simulink model "Simulation_File"  (R2017a)
settings: Solver=VariableStepAuto  StartTime=0.0  StopTime=50  FixedStep=Tsg  MaxStep=1e-3  RelTol=1e-3  EnableMultiTasking=on
InitFcn:
  | load('Wind_Perfil.mat')
  | 
  | Tsg=(1/5000);
  | TsPID=(1/5000);
  | TsWidfCV=0.01;
  | Ts=(1/5000);
  | 
  | %Parametros del convertidor
  | RD=0.01;
  | RQ=0.001;
  | RCi=0.01;
  | %RCi=0.1;
  | %RCi=1;
  | VD=0.7;
  | RL=0.1;
  | Ci=470e-6;
  | L=0.08;
  | Vdc_link=190.1681;
  | %Fs=5e3/1;
  | %Ts=1/Fs;
  | 
  | 
  | 
  | 
  | %% Battery Parameters
  | n_series = 50; % Number of series connected cells
  | n_parallel = 2; % Number of parallel branches
  | SOC_init = 0.5; % initial SOC
  | 
  | cell_cap = 6.5; % Cell capacitance
  | pack_cap = cell_cap * n_parallel; % Pack capacitance
  | 
  | cell_ConstI = 1.3; % Target constant charging current for each cell
  | cell_ConstV = 4.1; % Target constant charging voltage for each cell
  | 
  | ConstI = cell_ConstI * n_parallel; % Target constant charging current
  | ConstV = cell_ConstV * n_series; % Target constant charging voltage
  | 
  | MAX_SOC = 0.97; % State of charge when battery charging is stopped
  | 
  | %Parametros relacionados a sensado de corriente
  | G=100*1;
  | RG=1e3;
  | Rf=((G-1)*RG)/2;
  | DCR=RL;
  | Rcs=10e3;
  | Ccs=L/(DCR*Rcs);
undefined symbols (not defined in the file or in its folder): plecs
libraries: pil_lib x1
Description:
  | Software-in-the-Loop Code Verification
settings Model: ExtModeTrigDuration=10  ExtModeAutoUpdateStatusClock=off  Creator=The MathWorks, Inc.  LastModifiedBy=David R. LF
settings DataIOCC: SaveFormat=Array  SignalLogging=off  ReturnWorkspaceOutputs=on  SignalLoggingName=sigsOut
settings OptimizationCC: UseDivisionForNetSlopeComputation=UseDivisionForReciprocalsOfIntegersOnly  DefaultUnderspecifiedDataType=single  EnhancedBackFolding=on  BooleansAsBitfields=on  PassReuseOutputArgsAs=Individual arguments  ExpressionDepthLimit=2147483647  StateBitsets=on  DataBitsets=on  ZeroExternalMemoryAtStartup=off  NoFixptDivByZeroProtection=on  EfficientFloat2IntCast=on  LifeSpan=1  MaxStackSize=2560
settings DebuggingCC: CheckExecutionContextPreStartOutputMsg=on  CheckExecutionContextRuntimeOutputMsg=on  FcnCallInpInsideContextMsg=warning  AllowSymbolicDim=off  StateNameClashWarn=warning  StrictBusMsg=ErrorOnBusTreatedAsVector  SFUnexpectedBacktrackingDiag=warning  SFNoUnconditionalDefaultTransitionDiag=warning  SFExecutionAtInitializationDiag=none
settings HardwareCC: ProdBitPerPointer=32  ProdBitPerSizeT=32  ProdBitPerPtrDiffT=32  ProdLargestAtomicInteger=Long  ProdLargestAtomicFloat=Double  ProdWordSize=32  ProdLongLongMode=on  ProdHWDeviceType=ARM Compatible->ARM Cortex  TargetBitPerPointer=64  TargetBitPerSizeT=64  TargetBitPerPtrDiffT=64  TargetLongLongMode=on  TargetIntDivRoundTo=Zero  TargetEndianess=LittleEndian  TargetWordSize=64  TargetHWDeviceType=Generic->MATLAB Host Computer
settings ModelReferenceCC: PropagateSignalLabelsOutOfModel=off
settings SFSimCC: MATLABDynamicMemAlloc=off
settings RTWCC: SystemTargetFile=ert.tlc  HardwareBoard=TI Concerto F28M35x (ARM Cortex-M3)  TemplateMakefile=ert_default_tmf  Description=Embedded Coder  GenerateReport=on  RTWVerbose=off  Toolchain=Texas Instruments Code Composer Studio v6 (ARM)  IncludeHyperlinkInReport=on  CreateSILPILBlock=PIL  GenerateTraceInfo=on  GenerateTraceReport=on  GenerateTraceReportSl=on  GenerateTraceReportSf=on  GenerateTraceReportEml=on  GenerateCodeMetricsReport=on
settings CodeAppCC: ForceParamTrailComments=on  IgnoreCustomStorageClasses=off  IgnoreTestpoints=on  SimulinkDataObjDesc=on  CustomSymbolStrGlobalVar=rt$N$M  CustomSymbolStrType=$N$M  CustomSymbolStrFcn=$N$M$F  CustomSymbolStrMacro=$N$M  InsertBlockDesc=on  InternalIdentifier=Classic
settings ERTTargetCC: UtilityFuncGeneration=Shared location  MultiwordLength=2048  IncludeMdlTerminateFcn=off  CombineSignalStateStructs=on  SupportNonFinite=off  SupportContinuousTime=on  SupportVariableSizeSignals=on  ERTFilePackagingFormat=CompactWithDataFile  ConvertIfToSwitch=off  SuppressUnreachableDefaultCases=off
settings ConfigComp: CovMetricSettings=dw  CovHtmlReporting=on  CovSaveCumulativeToWorkspaceVar=on  CovSaveSingleToWorkspaceVar=on  CovExternalEMLEnable=off  CovSFcnEnable=off

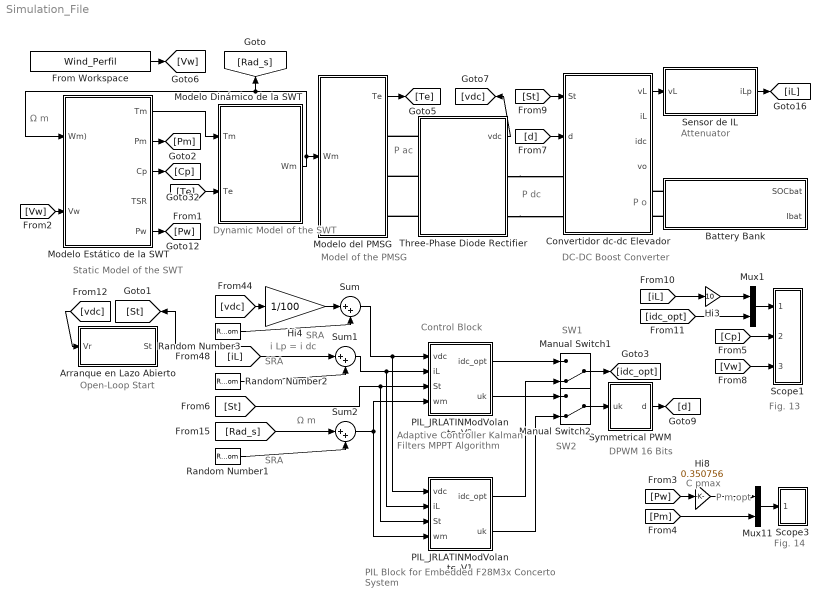
== system Simulation_File ==
  note: DPWM
      | 16 Bits
  note: i Lp = i dc
  note: Adaptive Controller
      | Kalman Filters
      | MPPT Algorithm
  note: Attenuator
  note: Open-Loop
      | Start
  note: DC-DC
      | Boost Converter
  note: P ac
  note: Model of
      | the PMSG
  note: Static Model
      | of the SWT
  note: Dynamic Model
      | of the SWT
  note: Ω m
  note: P dc
  note: P o
  note: SRA
  note: SRA
  note: Ω m
  note: SRA
  note: C pmax
  note: P m,opt
  note: Fig. 13
  note: Fig. 14
  note: PIL Block for Embedded F28M3x
      | Concerto System
  note: Control Block
  note: SW1
  note: SW2
  Arranque en Lazo Abierto : Subsystem  LoadFcn=plecs('sl', 200);  InitFcn=plecs('sl', 214);  StartFcn=plecs('sl', 208);  StopFcn=plecs('sl', 209);  mask(PlecsCircuit){PLECSData=<binary blob, 2632 chars, not shown>}
      mask prompts: PLECSData "PLECS Data (Do not delete or modify!)"
      mask init:
      | % PLACE CUSTOM INITIALIZATIONS ABOVE
      | % DO NOT REMOVE
      | plecs('sl', 215);
      | % DO NOT REMOVE
      settings: CopyFcn=plecs('sl', 203);  DeleteFcn=plecs('sl', 205);  UndoDeleteFcn=plecs('sl', 206);  PreSaveFcn=plecs('sl', 211);  PostSaveFcn=plecs('sl', 201);  NameChangeFcn=plecs('sl', 210);  DestroyFcn=plecs('sl', 207);  PreCopyFcn=plecs('sl', 216);  OpenFcn=plecs('sl', 202);  ErrorFcn=plerrorfcn
      mask Help: web(['file:///' fullfile(plecsdoc, 'creatingacircuit.html')])
      mask Display: disp('PLECS\nCircuit')
  Battery Bank : Subsystem  LoadFcn=plecs('sl', 200);  InitFcn=plecs('sl', 214);  StartFcn=plecs('sl', 208);  StopFcn=plecs('sl', 209);  mask(PlecsCircuit){PLECSData=<binary blob, 6620 chars, not shown>}
      mask prompts: PLECSData "PLECS Data (Do not delete or modify!)"
      mask init:
      | % PLACE CUSTOM INITIALIZATIONS ABOVE
      | % DO NOT REMOVE
      | plecs('sl', 215);
      | % DO NOT REMOVE
      settings: CopyFcn=plecs('sl', 203);  DeleteFcn=plecs('sl', 205);  UndoDeleteFcn=plecs('sl', 206);  PreSaveFcn=plecs('sl', 211);  PostSaveFcn=plecs('sl', 201);  NameChangeFcn=plecs('sl', 210);  DestroyFcn=plecs('sl', 207);  PreCopyFcn=plecs('sl', 216);  OpenFcn=plecs('sl', 202);  ErrorFcn=plerrorfcn
      mask Help: web(['file:///' fullfile(plecsdoc, 'creatingacircuit.html')])
      mask Display: disp('PLECS\nCircuit')
  Convertidor dc-dc Elevador : Subsystem  LoadFcn=plecs('sl', 200);  InitFcn=plecs('sl', 214);  StartFcn=plecs('sl', 208);  StopFcn=plecs('sl', 209);  mask(PlecsCircuit){PLECSData=<binary blob, 2184 chars, not shown>}
      mask prompts: PLECSData "PLECS Data (Do not delete or modify!)"
      mask init:
      | % PLACE CUSTOM INITIALIZATIONS ABOVE
      | % DO NOT REMOVE
      | plecs('sl', 215);
      | % DO NOT REMOVE
      settings: CopyFcn=plecs('sl', 203);  DeleteFcn=plecs('sl', 205);  UndoDeleteFcn=plecs('sl', 206);  PreSaveFcn=plecs('sl', 211);  PostSaveFcn=plecs('sl', 201);  NameChangeFcn=plecs('sl', 210);  DestroyFcn=plecs('sl', 207);  PreCopyFcn=plecs('sl', 216);  OpenFcn=plecs('sl', 202);  ErrorFcn=plerrorfcn
      mask Help: web(['file:///' fullfile(plecsdoc, 'creatingacircuit.html')])
      mask Display: disp('PLECS\nCircuit')
  From Workspace : FromWorkspace  VariableName=Wind_Perfil  SampleTime=1e-3
  Hi3 : Gain  Gain=10
  Hi4 : Gain  Gain=1/100
  Hi8 : Gain  Gain=0.350756
  Manual Switch1 : ManualSwitch  CurrentSetting=0
  Manual Switch2 : ManualSwitch  CurrentSetting=0
  Modelo del PMSG : Subsystem  LoadFcn=plecs('sl', 200);  InitFcn=plecs('sl', 214);  StartFcn=plecs('sl', 208);  StopFcn=plecs('sl', 209);  mask(PlecsCircuit){PLECSData=<binary blob, 5964 chars, not shown>}
      mask prompts: PLECSData "PLECS Data (Do not delete or modify!)"
      mask init:
      | % PLACE CUSTOM INITIALIZATIONS ABOVE
      | % DO NOT REMOVE
      | plecs('sl', 215);
      | % DO NOT REMOVE
      settings: CopyFcn=plecs('sl', 203);  DeleteFcn=plecs('sl', 205);  UndoDeleteFcn=plecs('sl', 206);  PreSaveFcn=plecs('sl', 211);  PostSaveFcn=plecs('sl', 201);  NameChangeFcn=plecs('sl', 210);  DestroyFcn=plecs('sl', 207);  PreCopyFcn=plecs('sl', 216);  OpenFcn=plecs('sl', 202);  ErrorFcn=plerrorfcn
      mask Help: web(['file:///' fullfile(plecsdoc, 'creatingacircuit.html')])
      mask Display: disp('PLECS\nCircuit')
  "Modelo Dinámico de la SWT " : Subsystem  LoadFcn=plecs('sl', 200);  InitFcn=plecs('sl', 214);  StartFcn=plecs('sl', 208);  StopFcn=plecs('sl', 209);  mask(PlecsCircuit){PLECSData=<binary blob, 2232 chars, not shown>}
      mask prompts: PLECSData "PLECS Data (Do not delete or modify!)"
      mask init:
      | % PLACE CUSTOM INITIALIZATIONS ABOVE
      | % DO NOT REMOVE
      | plecs('sl', 215);
      | % DO NOT REMOVE
      settings: CopyFcn=plecs('sl', 203);  DeleteFcn=plecs('sl', 205);  UndoDeleteFcn=plecs('sl', 206);  PreSaveFcn=plecs('sl', 211);  PostSaveFcn=plecs('sl', 201);  NameChangeFcn=plecs('sl', 210);  DestroyFcn=plecs('sl', 207);  PreCopyFcn=plecs('sl', 216);  OpenFcn=plecs('sl', 202);  ErrorFcn=plerrorfcn
      mask Help: web(['file:///' fullfile(plecsdoc, 'creatingacircuit.html')])
      mask Display: disp('PLECS\nCircuit')
  "Modelo Estático de la SWT " : Subsystem  LoadFcn=plecs('sl', 200);  InitFcn=plecs('sl', 214);  StartFcn=plecs('sl', 208);  StopFcn=plecs('sl', 209);  mask(PlecsCircuit){PLECSData=<binary blob, 3544 chars, not shown>}
      mask prompts: PLECSData "PLECS Data (Do not delete or modify!)"
      mask init:
      | % PLACE CUSTOM INITIALIZATIONS ABOVE
      | % DO NOT REMOVE
      | plecs('sl', 215);
      | % DO NOT REMOVE
      settings: CopyFcn=plecs('sl', 203);  DeleteFcn=plecs('sl', 205);  UndoDeleteFcn=plecs('sl', 206);  PreSaveFcn=plecs('sl', 211);  PostSaveFcn=plecs('sl', 201);  NameChangeFcn=plecs('sl', 210);  DestroyFcn=plecs('sl', 207);  PreCopyFcn=plecs('sl', 216);  OpenFcn=plecs('sl', 202);  ErrorFcn=plerrorfcn
      mask Help: web(['file:///' fullfile(plecsdoc, 'creatingacircuit.html')])
      mask Display: disp('PLECS\nCircuit')
  Mux1 : Mux  Inputs=2
  Mux11 : Mux  Inputs=2
  PIL_JRLATINModVolante_V1 : Subsystem  DialogController=pil_create_dialog  LoadFcn=|
      | try
      |    if ~strcmp(rtw.pil.getPILVersion, '6.12 (R2017a)_12')
      |       set_param(gcb, 'DialogController', '');
      |       set_param(gcb, 'DialogControllerArgs', '');
      |    end
      | catch e
      |       set_param(gcb, 'DialogController', '');
      |       set_param(gcb, 'DialogControllerArgs', '');
      | end
      mask help: PIL:pil:XILBlockMaskDesc
      mask Display: disp('PIL');
  PIL_JRLATINModVolante_V2 : Subsystem
  Random Number1 : RandomNumber  Variance=10*1  SampleTime=1e-3
  Random Number2 : RandomNumber  Variance=0.001*1  SampleTime=1e-3
  Random Number3 : RandomNumber  Variance=0.001*1  SampleTime=1e-3
  Scope1 : Subsystem  LoadFcn=plecs('sl', 300);  InitFcn=plecs('sl', 314);  StartFcn=plecs('sl', 308);  StopFcn=plecs('sl', 309);  mask{Settings=<binary blob, 1632 chars, not shown>}
      mask init:
      | plecs('sl', 315);
      settings: CopyFcn=plecs('sl', 303);  DeleteFcn=plecs('sl', 305);  UndoDeleteFcn=plecs('sl', 306);  PreSaveFcn=plecs('sl', 311);  NameChangeFcn=plecs('sl', 310);  DestroyFcn=plecs('sl', 307);  OpenFcn=plecs('sl', 302);  ErrorFcn=plerrorfcn
      mask Display: plot([0.1 0.9 0.9 0.1 0.1], [0.9 0.9 0.5 0.5 0.9])
  Scope3 : Subsystem  LoadFcn=plecs('sl', 300);  InitFcn=plecs('sl', 314);  StartFcn=plecs('sl', 308);  StopFcn=plecs('sl', 309);  mask{Settings=<binary blob, 1220 chars, not shown>}
      mask init:
      | plecs('sl', 315);
      settings: CopyFcn=plecs('sl', 303);  DeleteFcn=plecs('sl', 305);  UndoDeleteFcn=plecs('sl', 306);  PreSaveFcn=plecs('sl', 311);  NameChangeFcn=plecs('sl', 310);  DestroyFcn=plecs('sl', 307);  OpenFcn=plecs('sl', 302);  ErrorFcn=plerrorfcn
      mask Display: plot([0.1 0.9 0.9 0.1 0.1], [0.9 0.9 0.5 0.5 0.9])
  Sensor de IL : Subsystem  LoadFcn=plecs('sl', 200);  InitFcn=plecs('sl', 214);  StartFcn=plecs('sl', 208);  StopFcn=plecs('sl', 209);  mask(PlecsCircuit){PLECSData=<binary blob, 3020 chars, not shown>}
      mask prompts: PLECSData "PLECS Data (Do not delete or modify!)"
      mask init:
      | % PLACE CUSTOM INITIALIZATIONS ABOVE
      | % DO NOT REMOVE
      | plecs('sl', 215);
      | % DO NOT REMOVE
      settings: CopyFcn=plecs('sl', 203);  DeleteFcn=plecs('sl', 205);  UndoDeleteFcn=plecs('sl', 206);  PreSaveFcn=plecs('sl', 211);  PostSaveFcn=plecs('sl', 201);  NameChangeFcn=plecs('sl', 210);  DestroyFcn=plecs('sl', 207);  PreCopyFcn=plecs('sl', 216);  OpenFcn=plecs('sl', 202);  ErrorFcn=plerrorfcn
      mask Help: web(['file:///' fullfile(plecsdoc, 'creatingacircuit.html')])
      mask Display: disp('PLECS\nCircuit')
  Sum : Sum  Inputs=|++
  Sum1 : Sum  Inputs=|++
  Sum2 : Sum  Inputs=|++
  Symmetrical PWM : Subsystem  AncestorBlock=plecslib_extras2/Modulators/Symmetrical PWM  mask(Symmetrical PWM){sampling=Natural (carrier starts with 0), fc=5000, offset=0, input_limits=[0 65535], output_values=[0 1]}
      mask prompts: fc "Carrier frequency (Hz):"; offset "Carrier offset (p.u.):"; input_limits "Input limits [min max]:"; output_values "Output values [off on]:"
      mask help: PWM generator with a symmetrical triangular carrier. If the input is a vector, the output is also a vector of the same width.
      mask init:
      | if numel(fc)>1 || fc<=0,
      |   error('Carrier frequency must be a positive scalar.');
      | end
      | if numel(offset)>1 || offset<0 || offset>=1,
      |   error('Carrier offset must be a scalar in the range [0; 1/fc[.');
      | end
      | if sampling == 1,
      |   offset = mod(offset+.75, 1);
      | end
      | 
      | si = [.5 mod(offset, .5)]/fc;
      mask Help: eval('plecs(''help'', ''symmetricalpwm.html'')')
      mask TypeOptions sampling: Natural (carrier starts with 0) | Natural (carrier starts with 1) | Regular (double edge) | Regular (single edge)
  Three-Phase Diode Rectifier : Subsystem  LoadFcn=plecs('sl', 200);  InitFcn=plecs('sl', 214);  StartFcn=plecs('sl', 208);  StopFcn=plecs('sl', 209);  mask(PlecsCircuit){PLECSData=<binary blob, 1820 chars, not shown>}
      mask prompts: PLECSData "PLECS Data (Do not delete or modify!)"
      mask init:
      | % PLACE CUSTOM INITIALIZATIONS ABOVE
      | % DO NOT REMOVE
      | plecs('sl', 215);
      | % DO NOT REMOVE
      settings: CopyFcn=plecs('sl', 203);  DeleteFcn=plecs('sl', 205);  UndoDeleteFcn=plecs('sl', 206);  PreSaveFcn=plecs('sl', 211);  PostSaveFcn=plecs('sl', 201);  NameChangeFcn=plecs('sl', 210);  DestroyFcn=plecs('sl', 207);  PreCopyFcn=plecs('sl', 216);  OpenFcn=plecs('sl', 202);  ErrorFcn=plerrorfcn
      mask Help: web(['file:///' fullfile(plecsdoc, 'creatingacircuit.html')])
      mask Display: disp('PLECS\nCircuit')
  wires:
  Modelo del PMSG/1(Te) -> [Te]
  [St] -> Convertidor dc-dc Elevador/1(St)
  [d] -> Convertidor dc-dc Elevador/2(d)
  [Te] -> "Modelo Dinámico de la SWT "/2(Te)
  Three-Phase Diode Rectifier/1(vdc) -> [vdc]
  Sum/1 -> PIL_JRLATINModVolante_V1/1(vdc), PIL_JRLATINModVolante_V2/1(vdc)
  Sum1/1 -> PIL_JRLATINModVolante_V1/2(iL), PIL_JRLATINModVolante_V2/2(iL)
  [vdc] -> Arranque en Lazo Abierto/1(Vr)
  Arranque en Lazo Abierto/1(St) -> [St]
  [iL] -> Sum1/1
  Random Number2/1 -> Sum1/2
  Random Number3/1 -> Sum/2
  Sensor de IL/1(iLp) -> [iL]
  [St] -> PIL_JRLATINModVolante_V1/3(St), PIL_JRLATINModVolante_V2/3(St)
  "Modelo Estático de la SWT "/1(Tm) -> "Modelo Dinámico de la SWT "/1(Tm)
  "Modelo Dinámico de la SWT "/1(Wm) -> "Modelo Estático de la SWT "/1(Wm)), [Rad_s], Modelo del PMSG/1(Wm)
  [Vw] -> "Modelo Estático de la SWT "/2(Vw)
  Symmetrical PWM/1(d) -> [d]
  [Rad_s] -> Sum2/1
  Random Number1/1 -> Sum2/2
  Sum2/1 -> PIL_JRLATINModVolante_V1/4(wm), PIL_JRLATINModVolante_V2/4(wm)
  From Workspace/1 -> [Vw]
  Hi4/1 -> Sum/1
  [vdc] -> Hi4/1
  Convertidor dc-dc Elevador/1(vL) -> Sensor de IL/1(vL)
  "Modelo Estático de la SWT "/5(Pw) -> [Pw]
  [Pw] -> Hi8/1
  Hi8/1 -> Mux11/1
  Mux11/1 -> Scope3/1(1)
  "Modelo Estático de la SWT "/2(Pm) -> [Pm]
  [Pm] -> Mux11/2
  "Modelo Estático de la SWT "/3(Cp) -> [Cp]
  [Cp] -> Scope1/2(2)
  [Vw] -> Scope1/3(3)
  Mux1/1 -> Scope1/1(1)
  [idc_opt] -> Mux1/2
  [iL] -> Hi3/1
  Hi3/1 -> Mux1/1
  Manual Switch2/1 -> Symmetrical PWM/1(uk)
  PIL_JRLATINModVolante_V2/2(uk) -> Manual Switch2/1
  PIL_JRLATINModVolante_V2/1(idc_opt) -> Manual Switch1/1
  Manual Switch1/1 -> [idc_opt]
  PIL_JRLATINModVolante_V1/2(uk) -> Manual Switch2/2
  PIL_JRLATINModVolante_V1/1(idc_opt) -> Manual Switch1/2
  connections:
  Battery Bank/LConn1 -- Convertidor dc-dc Elevador/RConn1
  Three-Phase Diode Rectifier/LConn3 -- Modelo del PMSG/RConn3
  Three-Phase Diode Rectifier/LConn1 -- Modelo del PMSG/RConn1
  Three-Phase Diode Rectifier/RConn2 -- Convertidor dc-dc Elevador/LConn2
  Three-Phase Diode Rectifier/LConn2 -- Modelo del PMSG/RConn2
  Three-Phase Diode Rectifier/RConn1 -- Convertidor dc-dc Elevador/LConn1
  Battery Bank/LConn2 -- Convertidor dc-dc Elevador/RConn2

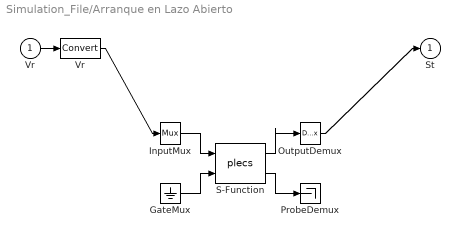
== system Simulation_File/Arranque en Lazo Abierto ==
  Vr : Inport  PortDimensions=1
  " GateMux " : Ground
  " InputMux " : Mux  Inputs=[ 1 ]
  " OutputDemux " : Demux  Outputs=[ 1 ]
  " ProbeDemux " : Terminator
  " S-Function " : S-Function  FunctionName=plecs  SFunctionDeploymentMode=off  EnableBusSupport=off
  " Vr " : DataTypeConversion  SaturateOnIntegerOverflow=on  RndMeth=Zero
  St : Outport  PortDimensions=1
  wires:
  " S-Function "/1 -> " OutputDemux "/1
  " InputMux "/1 -> " S-Function "/1
  " GateMux "/1 -> " S-Function "/2
  " S-Function "/2 -> " ProbeDemux "/1
  Vr/1 -> " Vr "/1
  " Vr "/1 -> " InputMux "/1
  " OutputDemux "/1 -> St/1

== system Simulation_File/Battery Bank ==
  +Vbat : PMIOPort  Port=1  Side=Left
  -Vbat : PMIOPort  Port=2  Side=Left
  SOCbat : Outport  PortDimensions=1
  Ibat : Outport  Port=2  PortDimensions=1
  wires:
  [PlecsSlave0Output1] -> SOCbat/1
  [PlecsSlave0Output2] -> Ibat/1

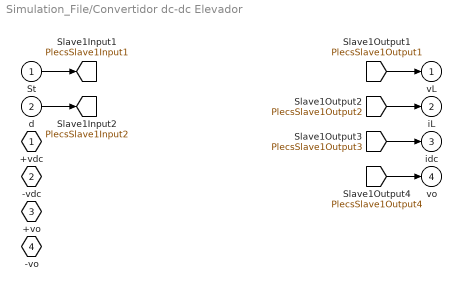
== system Simulation_File/Convertidor dc-dc Elevador ==
  St : Inport  PortDimensions=1
  d : Inport  Port=2  PortDimensions=1
  +vdc : PMIOPort  Port=1  Side=Left
  -vdc : PMIOPort  Port=2  Side=Left
  +vo : PMIOPort  Port=3  Side=Right
  -vo : PMIOPort  Port=4  Side=Right
  vL : Outport  PortDimensions=1
  iL : Outport  Port=2  PortDimensions=1
  idc : Outport  Port=3  PortDimensions=1
  vo : Outport  Port=4  PortDimensions=1
  tag scope: PlecsSlave1Input1=global, PlecsSlave1Input2=global
  wires:
  St/1 -> [PlecsSlave1Input1]
  [PlecsSlave1Output1] -> vL/1
  [PlecsSlave1Output2] -> iL/1
  [PlecsSlave1Output3] -> idc/1
  [PlecsSlave1Output4] -> vo/1
  d/1 -> [PlecsSlave1Input2]

== system Simulation_File/Modelo del PMSG ==
  Wm : Inport  PortDimensions=1
  va : PMIOPort  Port=1  Side=Right
  vb : PMIOPort  Port=2  Side=Right
  vc : PMIOPort  Port=3  Side=Right
  Te : Outport  PortDimensions=1
  tag scope: PlecsSlave2Input1=global
  wires:
  [PlecsSlave2Output1] -> Te/1
  Wm/1 -> [PlecsSlave2Input1]

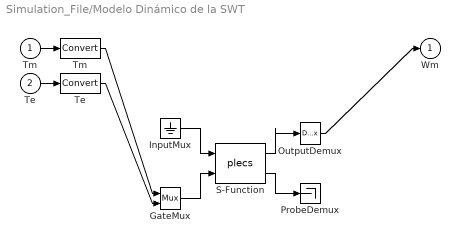
== system Simulation_File/Modelo Dinámico de la SWT  ==
  Tm : Inport  PortDimensions=1
  Te : Inport  Port=2  PortDimensions=1
  " GateMux " : Mux  Inputs=[ 1 1 ]
  " InputMux " : Ground
  " OutputDemux " : Demux  Outputs=[ 1 ]
  " ProbeDemux " : Terminator
  " S-Function " : S-Function  FunctionName=plecs  SFunctionDeploymentMode=off  EnableBusSupport=off
  " Te " : DataTypeConversion  SaturateOnIntegerOverflow=on  RndMeth=Zero
  " Tm " : DataTypeConversion  SaturateOnIntegerOverflow=on  RndMeth=Zero
  Wm : Outport  PortDimensions=1
  wires:
  " S-Function "/1 -> " OutputDemux "/1
  " InputMux "/1 -> " S-Function "/1
  " GateMux "/1 -> " S-Function "/2
  " S-Function "/2 -> " ProbeDemux "/1
  Tm/1 -> " Tm "/1
  " Tm "/1 -> " GateMux "/1
  Te/1 -> " Te "/1
  " Te "/1 -> " GateMux "/2
  " OutputDemux "/1 -> Wm/1

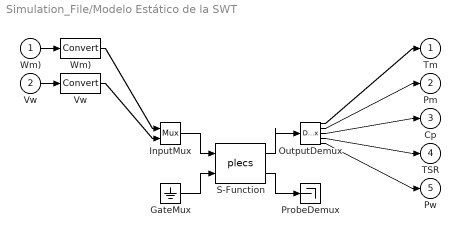
== system Simulation_File/Modelo Estático de la SWT  ==
  Wm) : Inport  PortDimensions=1
  Vw : Inport  Port=2  PortDimensions=1
  " GateMux " : Ground
  " InputMux " : Mux  Inputs=[ 1 1 ]
  " OutputDemux " : Demux  Outputs=[ 1 1 1 1 1 ]
  " ProbeDemux " : Terminator
  " S-Function " : S-Function  FunctionName=plecs  SFunctionDeploymentMode=off  EnableBusSupport=off
  " Vw " : DataTypeConversion  SaturateOnIntegerOverflow=on  RndMeth=Zero
  " Wm) " : DataTypeConversion  SaturateOnIntegerOverflow=on  RndMeth=Zero
  Tm : Outport  PortDimensions=1
  Pm : Outport  Port=2  PortDimensions=1
  Cp : Outport  Port=3  PortDimensions=1
  TSR : Outport  Port=4  PortDimensions=1
  Pw : Outport  Port=5  PortDimensions=1
  wires:
  " S-Function "/1 -> " OutputDemux "/1
  " InputMux "/1 -> " S-Function "/1
  " GateMux "/1 -> " S-Function "/2
  " S-Function "/2 -> " ProbeDemux "/1
  Wm)/1 -> " Wm) "/1
  " Wm) "/1 -> " InputMux "/1
  Vw/1 -> " Vw "/1
  " Vw "/1 -> " InputMux "/2
  " OutputDemux "/1 -> Tm/1
  " OutputDemux "/2 -> Pm/1
  " OutputDemux "/3 -> Cp/1
  " OutputDemux "/4 -> TSR/1
  " OutputDemux "/5 -> Pw/1

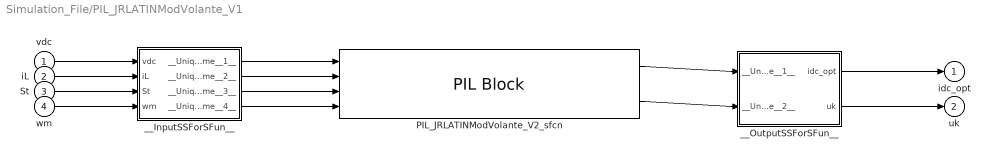
== system Simulation_File/PIL_JRLATINModVolante_V1 ==
  vdc : Inport
  iL : Inport  Port=2
  St : Inport  Port=3
  wm : Inport  Port=4
  PIL_JRLATINModVolante_V2_sfcn : pil_lib/PIL Block  SimulationMode=PIL  IsTopModelPIL=off  CodeDir=D:\PIL\F28M35XX_Cp_FESTO\PIL_JRLATINModVolante_V2_ert_rtw  ConfigName=Texas Instruments C2000 Concerto Serial  XrelIsTopModelCode=on
  __InputSSForSFun__ : Subsystem
  __OutputSSForSFun__ : Subsystem
  idc_opt : Outport
  uk : Outport  Port=2
  wires:
  vdc/1 -> __InputSSForSFun__/1(vdc)
  iL/1 -> __InputSSForSFun__/2(iL)
  St/1 -> __InputSSForSFun__/3(St)
  wm/1 -> __InputSSForSFun__/4(wm)
  __InputSSForSFun__/1(__UniqueOutportName__1__) -> PIL_JRLATINModVolante_V2_sfcn/1
  __InputSSForSFun__/2(__UniqueOutportName__2__) -> PIL_JRLATINModVolante_V2_sfcn/2
  __InputSSForSFun__/3(__UniqueOutportName__3__) -> PIL_JRLATINModVolante_V2_sfcn/3
  __InputSSForSFun__/4(__UniqueOutportName__4__) -> PIL_JRLATINModVolante_V2_sfcn/4
  PIL_JRLATINModVolante_V2_sfcn/1 -> __OutputSSForSFun__/1(__UniqueInportName__1__)
  PIL_JRLATINModVolante_V2_sfcn/2 -> __OutputSSForSFun__/2(__UniqueInportName__2__)
  __OutputSSForSFun__/1(idc_opt) -> idc_opt/1
  __OutputSSForSFun__/2(uk) -> uk/1

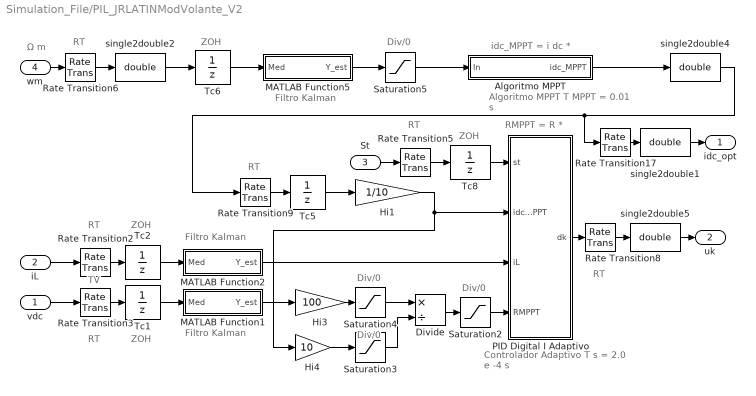
== system Simulation_File/PIL_JRLATINModVolante_V2 ==
  note: RT
  note: Div/0
  note: Filtro Kalman
  note: Ω m
  note: Algoritmo MPPT
      | T MPPT = 0.01 s
  note: ZOH
  note: idc_MPPT = i dc *
  note: ZOH
  note: RMPPT = R *
  note: Controlador Adaptivo
      | T s = 2.0 e -4 s
  note: Div/0
  note: Filtro Kalman
  note: Filtro Kalman
  note: ZOH
  note: ZOH
  note: Div/0
  note: Div/0
  note: TV
  note: RT
  note: RT
  note: RT
  note: RT
  note: RT
  vdc : Inport
  iL : Inport  Port=2
  St : Inport  Port=3
  wm : Inport  Port=4
  Algoritmo MPPT : MATLAB Function  TreatAsAtomicUnit=on
  Divide : Product  Inputs=*/
  Hi1 : Gain  Gain=1/10
  Hi3 : Gain  Gain=100
  Hi4 : Gain  Gain=10
  MATLAB Function1 : MATLAB Function  TreatAsAtomicUnit=on
  MATLAB Function2 : MATLAB Function  TreatAsAtomicUnit=on
  MATLAB Function5 : MATLAB Function  TreatAsAtomicUnit=on
  PID Digital I Adaptivo : MATLAB Function  TreatAsAtomicUnit=on
  Rate Transition{2..3,5,8..9,17} (6 alike) : RateTransition  OutPortSampleTime=TsPID
  Rate Transition6 : RateTransition  OutPortSampleTime=TsWidfCV
  Saturation2 : Saturate  UpperLimit=80  LowerLimit=5
  Saturation3 : Saturate  UpperLimit=15  LowerLimit=0.1
  Saturation4 : Saturate  UpperLimit=150  LowerLimit=10
  Saturation5 : Saturate  UpperLimit=300  LowerLimit=0.05
  Tc{1..2,5,8} (4 alike) : UnitDelay  SampleTime=TsPID
  Tc6 : UnitDelay  SampleTime=TsWidfCV
  single2double{1..2,4..5} (4 alike) : DataTypeConversion  OutDataTypeStr=double
  idc_opt : Outport
  uk : Outport  Port=2
  wires:
  Rate Transition8/1 -> single2double5/1
  Rate Transition9/1 -> Tc5/1
  Divide/1 -> Saturation2/1
  Hi3/1 -> Saturation4/1
  Hi4/1 -> Saturation3/1
  Rate Transition5/1 -> Tc8/1
  St/1 -> Rate Transition5/1
  Tc5/1 -> Hi1/1
  single2double5/1 -> uk/1
  Saturation3/1 -> Divide/2
  Saturation4/1 -> Divide/1
  Tc8/1 -> PID Digital I Adaptivo/1(st)
  PID Digital I Adaptivo/1(dk) -> Rate Transition8/1
  MATLAB Function2/1(Y_est) -> PID Digital I Adaptivo/3(iL)
  single2double2/1 -> Tc6/1
  wm/1 -> Rate Transition6/1
  Rate Transition6/1 -> single2double2/1
  Tc6/1 -> MATLAB Function5/1(Med)
  Saturation5/1 -> Algoritmo MPPT/1(In)
  MATLAB Function1/1(Y_est) -> Hi3/1
  Rate Transition3/1 -> Tc1/1
  Tc1/1 -> MATLAB Function1/1(Med)
  vdc/1 -> Rate Transition3/1
  Tc2/1 -> MATLAB Function2/1(Med)
  Rate Transition2/1 -> Tc2/1
  iL/1 -> Rate Transition2/1
  Hi1/1 -> Hi4/1, PID Digital I Adaptivo/2(idc_MPPT)
  single2double4/1 -> Rate Transition17/1, Rate Transition9/1
  Saturation2/1 -> PID Digital I Adaptivo/4(RMPPT)
  MATLAB Function5/1(Y_est) -> Saturation5/1
  Algoritmo MPPT/1(idc_MPPT) -> single2double4/1
  Rate Transition17/1 -> single2double1/1
  single2double1/1 -> idc_opt/1

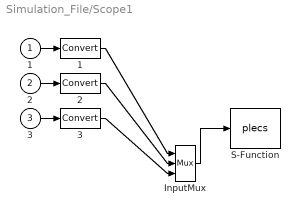
== system Simulation_File/Scope1 ==
  1 : Inport
  2 : Inport  Port=2
  3 : Inport  Port=3
  " 1 " : DataTypeConversion  SaturateOnIntegerOverflow=on  RndMeth=Zero
  " 2 " : DataTypeConversion  SaturateOnIntegerOverflow=on  RndMeth=Zero
  " 3 " : DataTypeConversion  SaturateOnIntegerOverflow=on  RndMeth=Zero
  " InputMux " : Mux  Inputs=3
  " S-Function " : S-Function  FunctionName=plecs  SFunctionDeploymentMode=off  EnableBusSupport=off
  wires:
  " InputMux "/1 -> " S-Function "/1
  1/1 -> " 1 "/1
  " 1 "/1 -> " InputMux "/1
  2/1 -> " 2 "/1
  " 2 "/1 -> " InputMux "/2
  3/1 -> " 3 "/1
  " 3 "/1 -> " InputMux "/3

== system Simulation_File/Scope3 ==
  1 : Inport
  " 1 " : DataTypeConversion  SaturateOnIntegerOverflow=on  RndMeth=Zero
  " InputMux " : Mux  Inputs=1
  " S-Function " : S-Function  FunctionName=plecs  SFunctionDeploymentMode=off  EnableBusSupport=off
  wires:
  " InputMux "/1 -> " S-Function "/1
  1/1 -> " 1 "/1
  " 1 "/1 -> " InputMux "/1

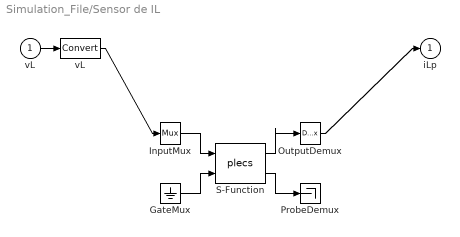
== system Simulation_File/Sensor de IL ==
  vL : Inport  PortDimensions=1
  " GateMux " : Ground
  " InputMux " : Mux  Inputs=[ 1 ]
  " OutputDemux " : Demux  Outputs=[ 1 ]
  " ProbeDemux " : Terminator
  " S-Function " : S-Function  FunctionName=plecs  SFunctionDeploymentMode=off  EnableBusSupport=off
  " vL " : DataTypeConversion  SaturateOnIntegerOverflow=on  RndMeth=Zero
  iLp : Outport  PortDimensions=1
  wires:
  " S-Function "/1 -> " OutputDemux "/1
  " InputMux "/1 -> " S-Function "/1
  " GateMux "/1 -> " S-Function "/2
  " S-Function "/2 -> " ProbeDemux "/1
  vL/1 -> " vL "/1
  " vL "/1 -> " InputMux "/1
  " OutputDemux "/1 -> iLp/1

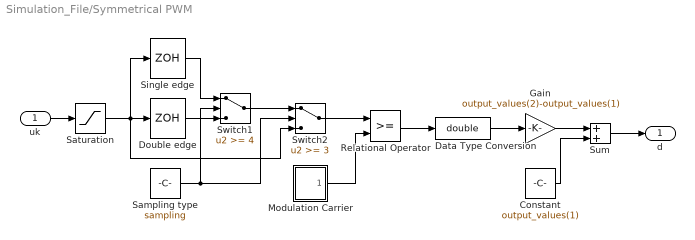
== system Simulation_File/Symmetrical PWM ==
  uk : Inport
  Constant : Constant  Value=output_values(1)
  Data Type Conversion : DataTypeConversion  OutDataTypeStr=double  SaturateOnIntegerOverflow=on  RndMeth=Zero
  Double edge : ZeroOrderHold  SampleTime=si
  Gain : Gain  Gain=output_values(2)-output_values(1)  SaturateOnIntegerOverflow=on  OutDataTypeStr=Inherit: Same as input  ParamDataTypeStr=Inherit: Same as input
  Modulation Carrier : Subsystem  mask(Symmetric Triangle Generator){fc=fc, offset=mod(offset+.5, 1), range=input_limits}
      mask prompts: fc "Carrier frequency (Hz):"; offset "Carrier offset (p.u.):"; range "Signal range [min max]:"
      mask help: Generates a symmetrical triangular signal with output values between 0 and 1. The block forces the Simulink solver to output all tips of the signal. The output can therefore be used as a carrier signal for PWM.
      mask init:
      | if numel(fc)>1 || fc<=0,
      |   error('Carrier frequency must be a positive scalar.');
      | end
      | if numel(offset)>1 || offset<0 || offset>=1,
      |   error('Carrier offset must be a scalar in the interval [0; 1[.');
      | end
      | if numel(range)~=2,
      |   error('Signal range must be a two-element vector.')
      | end
      | if range(1)>=range(2),
      |   error('Signal range must be specified as [min max].')
      | end
      | 
      | carrier_t = [0 offset mod(1/2+offset, 1) 1]/fc;
      | carrier_v0 = 1-2*abs(offset-.5);
      | carrier_v = range(1)+[carrier_v0 0 1 carrier_v0]*diff(range);
      | [carrier_t, idx] = unique(carrier_t);
      | carrier_v = carrier_v(idx);
      | si = [.5 mod(offset, .5)]/fc;
      | 
      | L = length(carrier_t);
      | disp_seq_t = repmat(carrier_t(:),1,3) + ones(L,1)*[0,1,2]/fc;
      | disp_seq_v = repmat(carrier_v(:),1,3);
      mask Display: plot(disp_seq_t, disp_seq_v)
  Relational Operator : RelationalOperator  RndMeth=Nearest  InputSameDT=on
  Sampling type : Constant  Value=sampling
  Saturation : Saturate  UpperLimit=input_limits(2)  LowerLimit=input_limits(1)
  Single edge : ZeroOrderHold  SampleTime=[1 offset]/fc
  Sum : Sum  SaturateOnIntegerOverflow=on  InputSameDT=on  OutDataTypeStr=Inherit: Same as first input
  Switch1 : Switch  Threshold=4  SaturateOnIntegerOverflow=on  InputSameDT=on
  Switch2 : Switch  Threshold=3  SaturateOnIntegerOverflow=on  InputSameDT=on
  d : Outport
  wires:
  Data Type Conversion/1 -> Gain/1
  Constant/1 -> Sum/2
  Gain/1 -> Sum/1
  Sum/1 -> d/1
  Relational Operator/1 -> Data Type Conversion/1
  Switch2/1 -> Relational Operator/1
  Sampling type/1 -> Switch1/2, Switch2/2
  Single edge/1 -> Switch1/1
  Saturation/1 -> Single edge/1, Switch2/3, Double edge/1
  uk/1 -> Saturation/1
  Modulation Carrier/1(Out) -> Relational Operator/2
  Switch1/1 -> Switch2/1
  Double edge/1 -> Switch1/3

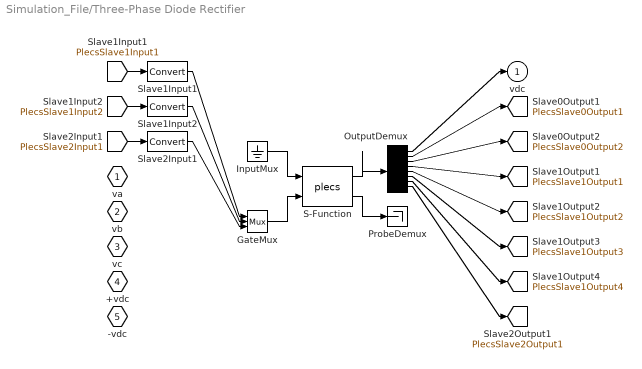
== system Simulation_File/Three-Phase Diode Rectifier ==
  "  Slave1Input1  " : DataTypeConversion  SaturateOnIntegerOverflow=on  RndMeth=Zero
  "  Slave1Input2  " : DataTypeConversion  SaturateOnIntegerOverflow=on  RndMeth=Zero
  "  Slave2Input1  " : DataTypeConversion  SaturateOnIntegerOverflow=on  RndMeth=Zero
  " GateMux " : Mux  Inputs=[ 1 1 1 ]
  " InputMux " : Ground
  " OutputDemux " : Demux  Outputs=[ 1 1 1 1 1 1 1 1 ]
  " ProbeDemux " : Terminator
  " S-Function " : S-Function  FunctionName=plecs  SFunctionDeploymentMode=off  EnableBusSupport=off
  va : PMIOPort  Port=1  Side=Left
  vb : PMIOPort  Port=2  Side=Left
  vc : PMIOPort  Port=3  Side=Left
  +vdc : PMIOPort  Port=4  Side=Right
  -vdc : PMIOPort  Port=5  Side=Right
  vdc : Outport  PortDimensions=1
  tag scope: PlecsSlave0Output1=global, PlecsSlave0Output2=global, PlecsSlave1Output1=global, PlecsSlave1Output2=global, PlecsSlave1Output3=global, PlecsSlave1Output4=global, PlecsSlave2Output1=global
  wires:
  " S-Function "/1 -> " OutputDemux "/1
  " InputMux "/1 -> " S-Function "/1
  " GateMux "/1 -> " S-Function "/2
  " S-Function "/2 -> " ProbeDemux "/1
  [PlecsSlave1Input1] -> "  Slave1Input1  "/1
  "  Slave1Input1  "/1 -> " GateMux "/1
  [PlecsSlave1Input2] -> "  Slave1Input2  "/1
  "  Slave1Input2  "/1 -> " GateMux "/2
  [PlecsSlave2Input1] -> "  Slave2Input1  "/1
  "  Slave2Input1  "/1 -> " GateMux "/3
  " OutputDemux "/1 -> vdc/1
  " OutputDemux "/2 -> [PlecsSlave0Output1]
  " OutputDemux "/3 -> [PlecsSlave0Output2]
  " OutputDemux "/4 -> [PlecsSlave1Output1]
  " OutputDemux "/5 -> [PlecsSlave1Output2]
  " OutputDemux "/6 -> [PlecsSlave1Output3]
  " OutputDemux "/7 -> [PlecsSlave1Output4]
  " OutputDemux "/8 -> [PlecsSlave2Output1]

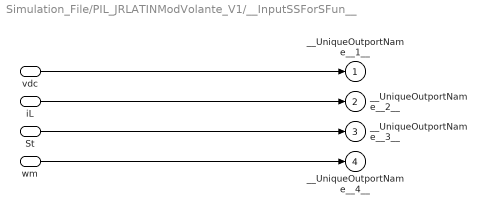
== system Simulation_File/PIL_JRLATINModVolante_V1/__InputSSForSFun__ ==
  vdc : Inport
  iL : Inport  Port=2
  St : Inport  Port=3
  wm : Inport  Port=4
  __UniqueOutportName__1__ : Outport
  __UniqueOutportName__2__ : Outport  Port=2
  __UniqueOutportName__3__ : Outport  Port=3
  __UniqueOutportName__4__ : Outport  Port=4
  wires:
  vdc/1 -> __UniqueOutportName__1__/1
  iL/1 -> __UniqueOutportName__2__/1
  St/1 -> __UniqueOutportName__3__/1
  wm/1 -> __UniqueOutportName__4__/1

== system Simulation_File/PIL_JRLATINModVolante_V1/__OutputSSForSFun__ ==
  __UniqueInportName__1__ : Inport
  __UniqueInportName__2__ : Inport  Port=2
  idc_opt : Outport
  uk : Outport  Port=2
  wires:
  __UniqueInportName__1__/1 -> idc_opt/1
  __UniqueInportName__2__/1 -> uk/1

== system Simulation_File/Symmetrical PWM/Modulation Carrier ==
  Clock : Clock
  Fcn : Fcn  Expr=u*fc-offset
  Lookup Table : Lookup  InputValues=[0 .5 1]  Table=[range(1) range(2) range(1)]  LookUpMeth=Interpolation-Use End Values
  Rounding Function : Rounding
  Subtract : Sum  Inputs=+-
  Unit Delay : UnitDelay  SampleTime=si
  Out : Outport
  wires:
  Lookup Table/1 -> Out/1
  Subtract/1 -> Lookup Table/1
  Rounding Function/1 -> Subtract/2
  Fcn/1 -> Rounding Function/1, Subtract/1
  Clock/1 -> Fcn/1
  Unit Delay/1 -> Unit Delay/1

== matlab function Simulation_File/PIL_JRLATINModVolante_V2/MATLAB Function2 ==
  data: Med input; Y_est output
function Y_est   = fcn(Med)
persistent Q R K P_temp x_temp_est P X_est P_ant X_est_ant
if isempty(K)
Q = 0.001;
R = 10;
K =0;
P_temp=0;
x_temp_est=0;
P_ant=0;
X_est_ant=0;
P=0;
X_est=0;
end
  x_temp_est = X_est_ant; 
  P_temp = P_ant + Q;
  K = P_temp * (1.0/(P_temp + R));
  X_est = x_temp_est + K * (Med - x_temp_est); 
  P = (1- K) * P_temp;
  P_ant=P;
  X_est_ant=X_est;
  Y_est=X_est;
end

== matlab function Simulation_File/PIL_JRLATINModVolante_V2/Algoritmo MPPT ==
  data: In input; idc_MPPT output
function idc_MPPT   = fcn(In)
Ir_Interpolacion=[0.0746 0.252 0.562 0.877 1.21 1.73 2.22 2.87 3.52 4.31 5.23 6.13 7.23 8.35 9.8 1.11 1.27 1.43 1.61];
V_wInterpolacion=[2 3 4 5 6 7 8 9 10 11 12 13 14 15 16 17 18 19 20];
Wm_Interpolacion=[23.5 31.2 39.6 51.7 63.1 73.9 84.6 95.1 104 116 126 138 148 159 170 180 191 203 213];




idc_MPPT=interp1(Wm_Interpolacion,Ir_Interpolacion,In,'linear');
%idc_MPPT=interp1(V_wInterpolacion,Ir_Interpolacion,In,'linear');

end

== matlab function Simulation_File/PIL_JRLATINModVolante_V2/MATLAB Function5 ==
  data: Med input; Y_est output
function Y_est   = fcn(Med)
persistent Q R K P_temp x_temp_est P X_est P_ant X_est_ant
if isempty(K)
Q = 0.1;
R = 10;
K =0;
P_temp=0;
x_temp_est=0;
P_ant=0;
X_est_ant=0;
P=0;
X_est=0;
end
  x_temp_est = X_est_ant; 
  P_temp = P_ant + Q;
  K = P_temp * (1.0/(P_temp + R));
  X_est = x_temp_est + K * (Med - x_temp_est); 
  P = (1- K) * P_temp;
  P_ant=P;
  X_est_ant=X_est;
  Y_est=X_est;
end

== matlab function Simulation_File/PIL_JRLATINModVolante_V2/MATLAB Function1 ==
  data: Med input; Y_est output
function Y_est   = fcn(Med)
persistent Q R K P_temp x_temp_est P X_est P_ant X_est_ant
if isempty(K)
Q = 0.0001;
R = 10;
K =0;
P_temp=0;
x_temp_est=0;
P_ant=0;
X_est_ant=0;
P=0;
X_est=0;
end
  x_temp_est = X_est_ant; 
  P_temp = P_ant + Q;
  K = P_temp * (1.0/(P_temp + R));
  X_est = x_temp_est + K * (Med - x_temp_est); 
  P = (1- K) * P_temp;
  P_ant=P;
  X_est_ant=X_est;
  Y_est=X_est;
end

== matlab function Simulation_File/PIL_JRLATINModVolante_V2/PID Digital I Adaptivo ==
  data: st input; dk output; idc_MPPT input; iL input; RMPPT input
function dk  = fcn(st, idc_MPPT, iL, RMPPT)

 %Valores iniciales de las constantes del controlador
 persistent  ni1 ni2 ni3 di2 di3
 persistent  eik uik
 persistent  eik_1 eik_2 uik_1 uik_2
 if isempty(eik)
    ni1=2.7571e+05;
    ni2=-5.4173e+05;
    ni3=2.6611e+05;
    di2=-1.9659; 
    di3=0.9659;
    eik =0;
    uik =0;
    eik_1 =0;
    eik_2 =0;
    uik_1 =0;
    uik_2 =0;
 end
    
%Frecuencia de muestreo
Ts=(1/5000);
%Parametros del convertidor cd-cd elevador
RD=0.00;
RQ=0.000;
VD=0.0;
RL=0.0;
Ci=470e-6;
L=0.08;
Vdc=190.1681;
if(st==1)
%Controlador PID digital para corriente
m=0.5;
b=16;
RCi=0.00;
Kpwm=1/(2^b-1);
A=(Kpwm*Vdc)/L;
B=(Kpwm*Vdc)/(Ci*L*RMPPT);
a=(L-sqrt(complex(L^2-4*Ci*L*RMPPT^2)))/(2*Ci*L*RMPPT);
b=(L+sqrt(complex(L^2-4*Ci*L*RMPPT^2)))/(2*Ci*L*RMPPT);
C=(A/(b-a))*(exp(-Ts*a*m)-exp(-Ts*b*m));
e1=(exp(-Ts*a)*exp(-Ts*b*m)-exp(-Ts*b)*exp(-Ts*a*m))/(exp(-Ts*a*m)-exp(-Ts*b*m));
D=B*(a-b-a*exp(-Ts*b*m)+b*exp(-Ts*a*m))/(a*b*(a-b));
c=(b*exp(-Ts*a)-a*exp(-Ts*b)-a*exp(-Ts*a)+b*exp(-Ts*b)+a*exp(-Ts*b*m)-b*exp(-Ts*a*m)+a*exp(-Ts*a)*exp(-Ts*b*m)-b*exp(-Ts*b)*exp(-Ts*a*m)+sqrt((b*exp(-Ts*a)-a*exp(-Ts*b)-a*exp(-Ts*a)+b*exp(-Ts*b)+a*exp(-Ts*b*m)-b*exp(-Ts*a*m)+a*exp(-Ts*a)*exp(-Ts*b*m)-b*exp(-Ts*b)*exp(-Ts*a*m))^2+4*(a*exp(-Ts*a)*exp(-Ts*b*m)-b*exp(-Ts*b)*exp(-Ts*a*m)-a*exp(-Ts*a)*exp(-Ts*b)+b*exp(-Ts*a)*exp(-Ts*b))*(a-b-a*exp(-Ts*b*m)+b*exp(-Ts*a*m))))/(2*(a-b-a*exp(-Ts*b*m)+b*exp(-Ts*a*m)));
d=(b*exp(-Ts*a)-a*exp(-Ts*b)-a*exp(-Ts*a)+b*exp(-Ts*b)+a*exp(-Ts*b*m)-b*exp(-Ts*a*m)+a*exp(-Ts*a)*exp(-Ts*b*m)-b*exp(-Ts*b)*exp(-Ts*a*m)-sqrt((b*exp(-Ts*a)-a*exp(-Ts*b)-a*exp(-Ts*a)+b*exp(-Ts*b)+a*exp(-Ts*b*m)-b*exp(-Ts*a*m)+a*exp(-Ts*a)*exp(-Ts*b*m)-b*exp(-Ts*b)*exp(-Ts*a*m))^2+4*(a*exp(-Ts*a)*exp(-Ts*b*m)-b*exp(-Ts*b)*exp(-Ts*a*m)-a*exp(-Ts*a)*exp(-Ts*b)+b*exp(-Ts*a)*exp(-Ts*b))*(a-b-a*exp(-Ts*b*m)+b*exp(-Ts*a*m))))/(2*(a-b-a*exp(-Ts*b*m)+b*exp(-Ts*a*m)));
g=real((D*c-C+D*d+C*e1-sqrt(C^2*e1^2+2*C^2*e1+C^2-4*C*D*c*d+2*C*D*c*e1-2*C*D*c+2*C*D*d*e1-2*C*D*d+4*C*D*e1+D^2*c^2-2*D^2*c*d+D^2*d^2))/(2*(C+D)));
h=real((D*c-C+D*d+C*e1+sqrt(C^2*e1^2+2*C^2*e1+C^2-4*C*D*c*d+2*C*D*c*e1-2*C*D*c+2*C*D*d*e1-2*C*D*d+4*C*D*e1+D^2*c^2-2*D^2*c*d+D^2*d^2))/(2*(C+D)));
%Disenamos controlador digitial PID con filtro basado en Gidz2
deltaGainPID=1;
deltaZ1=1;
deltaZ2=1;
deltaP1=1;
PID_G=((1/(C+D)-((1-deltaGainPID)*(1/(C+D)))));
PID_Z1=((abs(real(exp(-Ts*a)))-((1-deltaZ1)*(abs(real(exp(-Ts*a)))))));
PID_Z2=(((abs(real(exp(-Ts*b)))-((1-deltaZ2)*(abs(real(exp(-Ts*b))))))));
PID_P1=abs(h);
PID_P2=((abs(g)-((1-deltaP1)*(abs(g)))));
%Calculo de parametros de controlador de corriente
ni1=PID_G;
ni2= -PID_G*PID_Z1 - PID_G*PID_Z2;
ni3= PID_G*PID_Z1*PID_Z2;
di1= 1;
di2=-PID_P1-PID_P2;
di3= PID_P1*PID_P2;


eik=idc_MPPT-iL;
uik=real(ni1*eik+ni2*eik_1+ni3*eik_2-di2*uik_1-di3*uik_2);
uik(isnan(uik))=0;
eik_2=eik_1;
eik_1=eik;
uik_2=uik_1;
uik_1=uik;
if(uik<0)
uik=0;
end
if(uik>65536)
uik=65536;
end
dk=uik;
else
dk =0;  
eik=0;
uik=0;
end
